simulink library "simulink_lib_MDB"  (R2015a)
settings: Solver=ode45  StartTime=0.0  StopTime=10.0  RelTol=1e-3
settings Model: Creator=mainster  LastModifiedBy=mainster
settings DebuggingCC: UnderspecifiedInitializationDetection=Classic  MergeDetectMultiDrivingBlocksExec=none  SolverPrmCheckMsg=warning  StateNameClashWarn=warning

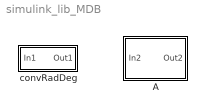
== system simulink_lib_MDB ==
  A : Subsystem  mask{MNAME=A, MMAT=[[1,2];[3,4]], SampleTime=-1, mskcont=on, doUpdate=on}
      mask prompts: MNAME "Matrix Name:"; MMAT "Matrix / Vector / scalar Gain"; SampleTime "Sample time (-1 for inherited):"; mskcont "draw matrix / vector to mask?"; doUpdate "auto update diagram?"
      mask init:
      | %SampleTime=-1
      | %MNAME='A'
      | %MMAT=[[1,2];[3,4]]
      | %sMMAT=size(MMAT)
      | %UPDATE=0;
      settings: CopyFcn=|
      | h=get_param(gcb,'Name');
      | ind=regexp(h,'[0-9]*\.?[0-9]*');
      | 
      | blocks='none';
      | CNT=str2num(h(ind(1)))+1;
      | 
      | 
      | while ~isempty(blocks)
      |   blocks = find_system(gcs,'Type','Block','Name',...
      |             [h(1:ind(1)-1); num2str(str2num(h(ind(1)))+CNT)]);
      | CNT=CNT+1;
      | end
      | 
      | nn=[h(1:ind(1)-1); num2str(str2num(h(ind(1)))+CNT-1)];
      |  set_param(gcb,'MNAME',nn);
      |  set_param(gcb,'Name',nn);
      settings: NameChangeFcn=|
      | new=get_param(gcb,'Name');
      | set_param(gcb,'MNAME',new);
      mask TypeOptions MMAT: Gain3/Gain
      mask Callback MMAT:
      | doUpdate = get_param(gcb,'doUpdate');
      | if doUpdate == true
      | %   disp('update');
      |    set_param(gcs, 'SimulationCommand', 'update');
      | else
      | %   disp(new);
      | end
      mask TypeOptions SampleTime: Gain3/SampleTime
      mask Callback mskcont: %eval(mskcont);
      mask Callback doUpdate:
      | %eval(UPDATE);
      | %sprintf('%s',UPDATE)
      | %UPDATE
      mask Display:
      | h=get_param(gcb,'handle');
      | set(h,'Name',MNAME);
      | if mskcont==false
      |     disp([MNAME]);
      |     set(h,'ShowName','off');
      | else
      |     str=[];
      |     for k=1:size(MMAT,1)
      |         str=[ str '\n' '[' num2str(MMAT(k,:)) ']'];
      |     end
      |     disp(str(3:end));
      |     set(h,'ShowName','on');
      | end
  convRadDeg : Subsystem  mask{r2d=on, tmp=180/pi}
      mask prompts: r2d "Radian to Degree"; tmp "Gain:"
      mask Callback r2d:
      | if strcmpi(get_param(gcb, 'r2d'),'on')
      |     set_param(gcb,'tmp',num2str(180/pi))
      | else
      |     set_param(gcb,'tmp',num2str(pi/180))
      | end
      mask TypeOptions tmp: deg2rad1/Gain
      mask Display:
      | if r2d
      |     fprintf('Rad2Deg')
      | else
      |     fprintf('Deg2Rad')
      | end

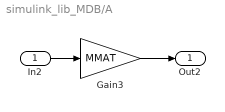
== system simulink_lib_MDB/A ==
  In2 : Inport
  Gain3 : Gain  Gain=MMAT  SampleTime=SampleTime
  Out2 : Outport
  wires:
  In2/1 -> Gain3/1
  Gain3/1 -> Out2/1

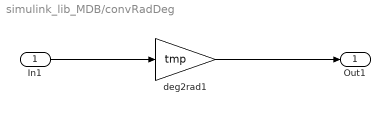
== system simulink_lib_MDB/convRadDeg ==
  In1 : Inport
  deg2rad1 : Gain  Gain=tmp
  Out1 : Outport
  wires:
  In1/1 -> deg2rad1/1
  deg2rad1/1 -> Out1/1
